simulink model "invPendStateFeedback"  (R2019a)
settings: Solver=ode45  StartTime=0.0  StopTime=5  RelTol=1e-6
values from neighbouring files (symbols this model uses):
  A = [0       1            0         0 ... (first row only)    [pendulumParameters.m]
  B = [    0 ... (first row only)    [pendulumParameters.m]
  C = eye(4)    [pendulumParameters.m]
  D = [0 ... (first row only)    [pendulumParameters.m]
  K = place(A,B,[-5,-4,-3,-2])    [pendulumStateFeedback.m]
  x0 = [0 0 theta0 0]'    [pendulumStateFeedback.m]
settings Model: Creator=alfredo  LastModifiedBy=adria
settings DataIOCC: ReturnWorkspaceOutputs=off
settings DebuggingCC: ArithmeticOperatorsInVariantConditions=warning
settings SFSimCC: SimUseLocalCustomCode=off
settings RTWCC: RTWUseLocalCustomCode=off

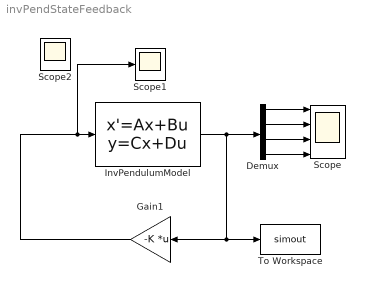
== system invPendStateFeedback ==
  Demux : Demux  Outputs=[1 1 1 1]
  Gain1 : Gain  Gain=-K  Multiplication=Matrix(K*u)
  InvPendulumModel : StateSpace  A=A  B=B  C=C  D=D  InitialCondition=x0
  Scope : Scope  NumInputPorts=4
  Scope1 : Scope
  To Workspace : ToWorkspace  VariableName=simout  SaveFormat=Structure With Time  SampleTime=-1
  Scope2 : Scope
  wires:
  Gain1/1 -> Scope1/1, InvPendulumModel/1
  InvPendulumModel/1 -> Gain1/1, To Workspace/1, Demux/1
  Demux/1 -> Scope/1
  Demux/2 -> Scope/2
  Demux/3 -> Scope/3
  Demux/4 -> Scope/4
